simulink library "CassieLibrary"  (R2017b)
settings: Solver=VariableStepAuto  StartTime=0.0  StopTime=10.0  RelTol=1e-3
undefined symbols (not defined in the file): DiagnosticCodes, motorPositions, motorVelocities, X, Y, Z
libraries: sm_lib x50, ComponentLibrary x19, xpcethercatlib x15, CassieLibrary x10, xpcutilitieslib x2, simulink x2, Contact_Forces_Lib x2, nesl_utility x2, slrtlib x1
(part 1 of 3)
settings Model: Creator=Mikhail  LastModifiedBy=jreher

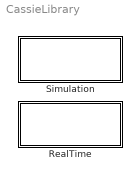
== system CassieLibrary ==
  RealTime : Subsystem
  Simulation : Subsystem

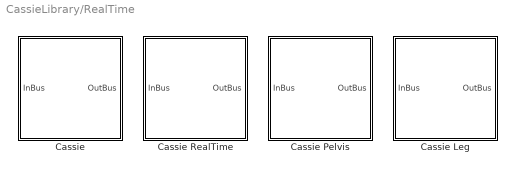
== system CassieLibrary/RealTime ==
  Cassie : Subsystem  InitFcn=|
      | % Import bus definitions
      | CassieModule.importBuses;
      mask Display: image('Cassie.png');
  Cassie Leg : Subsystem  mask{config=Left}
      mask prompts: config "Configuration:"
      mask init:
      | switch config
      |   case 1 % Left
      |     set_param([gcb, '/Hip Roll Drive'], 'ethercatName', 'Left Hip Roll Drive');
      |     set_param([gcb, '/Hip Roll Drive'], 'slaveAddress', '1002');
      |     set_param([gcb, '/Hip Yaw Drive'], 'ethercatName', 'Left Hip Yaw Drive');
      |     set_param([gcb, '/Hip Yaw Drive'], 'slaveAddress', '1003');
      |     set_param([gcb, '/Hip Pitch Drive'], 'ethercatName', 'Left Hip Pitch Drive');
      |     set_param([gcb, '/Hip Pitch Drive'], 'slaveAddress', '1004');
      |     set_param([gcb, '/Knee Drive'], 'ethercatName', 'Left Knee Drive');
      |     set_param([gcb, '/Knee Drive'], 'slaveAddress', '1005');
      |     set_param([gcb, '/Foot Drive'], 'ethercatName', 'Left Foot Drive');
      |     set_param([gcb, '/Foot Drive'], 'slaveAddress', '1006');
      |     set_param([gcb, '/Counter PDO Receive'], 'sig_name', 'Left Leg Medulla.Base Inputs.Counter');
      |     set_param([gcb, '/CPU Load PDO Receive'], 'sig_name', 'Left Leg Medulla.Base Inputs.CPU Load');
      |     set_param([gcb, '/Reed Switch State PDO Receive'], 'sig_name', 'Left Leg Medulla.Misc Inputs.Reed Switch');
      |     set_param([gcb, '/Shin Joint Encoder PDO Receive'], 'sig_name', 'Left Leg Medulla.Misc Inputs.Knee Spring Encoder');
      |     set_param([gcb, '/Tarsus Joint Encoder PDO Receive'], 'sig_name', 'Left Leg Medulla.Misc Inputs.Ankle Joint Encoder');
      |     set_param([gcb, '/Foot Joint Encoder PDO Receive'], 'sig_name', 'Left Leg Medulla.Misc Inputs.Foot Joint Encoder');
      |     set_param([gcb, '/Shin Joint Encoder Gain'], 'Gain', '-1/2^19*2*pi');
      |     set_param([gcb, '/Tarsus Joint Encoder Gain'], 'Gain', '-1/2^19*2*pi');
      |     set_param([gcb, '/Foot Joint Encoder Gain'], 'Gain', '-1/2^13*2*pi');
      |     
      |   case 2 % Right
      |     set_param([gcb, '/Hip Roll Drive'], 'ethercatName', 'Right Hip Roll Drive');
      |     set_param([gcb, '/Hip Roll Drive'], 'slaveAddress', '1008');
      |     set_param([gcb, '/Hip Yaw Drive'], 'ethercatName', 'Right Hip Yaw Drive');
      |     set_param([gcb, '/Hip Yaw Drive'], 'slaveAddress', '1009');
      |     set_param([gcb, '/Hip Pitch Drive'], 'ethercatName', 'Right Hip Pitch Drive');
      |     set_param([gcb, '/Hip Pitch Drive'], 'slaveAddress', '1012');
      |     set_param([gcb, '/Knee Drive'], 'ethercatName', 'Right Knee Drive');
      |     set_param([gcb, '/Knee Drive'], 'slaveAddress', '1011');
      |     set_param([gcb, '/Foot Drive'], 'ethercatName', 'Right Foot Drive');
      |     set_param([gcb, '/Foot Drive'], 'slaveAddress', '1010');
      |     set_param([gcb, '/Counter PDO Receive'], 'sig_name', 'Right Leg Medulla.Base Inputs.Counter');
      |     set_param([gcb, '/CPU Load PDO Receive'], 'sig_name', 'Right Leg Medulla.Base Inputs.CPU Load');
      |     set_param([gcb, '/Reed Switch State PDO Receive'], 'sig_name', 'Right Leg Medulla.Misc Inputs.Reed Switch');
      |     set_param([gcb, '/Shin Joint Encoder PDO Receive'], 'sig_name', 'Right Leg Medulla.Misc Inputs.Knee Spring Encoder');
      |     set_param([gcb, '/Tarsus Joint Encoder PDO Receive'], 'sig_name', 'Right Leg Medulla.Misc Inputs.Ankle Joint Encoder');
      |     set_param([gcb, '/Foot Joint Encoder PDO Receive'], 'sig_name', 'Right Leg Medulla.Misc Inputs.Foot Joint Encoder');
      |     set_param([gcb, '/Shin Joint Encoder Gain'], 'Gain', '1/2^19*2*pi');
      |     set_param([gcb, '/Tarsus Joint Encoder Gain'], 'Gain', '1/2^19*2*pi');
      |     set_param([gcb, '/Foot Joint Encoder Gain'], 'Gain', '1/2^13*2*pi');
      | end % switch
      | 
      | % Check if block is not in library model
      | if ~bdIsLibrary(bdroot)
      |   % Construct discrete filter for velocity estimation
      |   dt = str2num(get_param(bdroot, 'FixedStep'));
      |   filter1 = ButterworthFilter(2);
      |   filter1.setTimeConstant(0.003, dt);
      |   filter2 = BackwardDifferencingFilter(2);
      |   filter2.setSampleTime(dt);
      |   filter3 = Filter(filter1, filter2, 'cascade');
      |   [a, b] = filter3.getCoefficients;
      |   
      |   % Set discrete filter coefficients    
      |   set_param([gcb '/Shin Filter'], 'a', mat2str(a));
      |   set_param([gcb '/Shin Filter'], 'b', mat2str(b));
      |   set_param([gcb '/Tarsus Filter'], 'a', mat2str(a));
      |   set_param([gcb '/Tarsus Filter'], 'b', mat2str(b));
      |   set_param([gcb '/Foot Filter'], 'a', mat2str(a));
      |   set_param([gcb '/Foot Filter'], 'b', mat2str(b));
      | end % if
      settings: PermitHierarchicalResolution=None
      mask TypeOptions config: Left | Right
  Cassie Pelvis : Subsystem
      settings: PermitHierarchicalResolution=None
  Cassie RealTime : Subsystem
      settings: PermitHierarchicalResolution=None
      mask Display: image('Cassie.png');

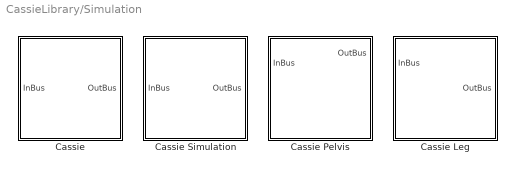
== system CassieLibrary/Simulation ==
  Cassie : Subsystem  InitFcn=|  StartFcn=|  StopFcn=|
      InitFcn=|
      | % Start clock at initialization (used for computing real time performance)
      | initTime = tic;
      | 
      | % Import bus definitions
      | CassieModule.importBuses;
      StartFcn=|
      | % Store build time
      | buildTime = toc(initTime);
      StopFcn=|
      | % Store computation time
      | computationTime = toc(initTime) - buildTime;
      | 
      | % Get simulation time
      | simulationTime = get_param(bdroot, 'SimulationTime');
      | 
      | % Compute real time performance
      | percentRealTime = 100*simulationTime/computationTime;
      | 
      | % Display
      | fprintf('Build time: %0.2f seconds \n', buildTime);
      | fprintf('Simulation time: %0.2f seconds \n', simulationTime);
      | fprintf('Computation time: %0.2f seconds \n', computationTime);
      | fprintf('Performance: %0.2f%% real time \n', percentRealTime);
      mask Display: image('Cassie.png');
  Cassie Leg : Subsystem  mask{config=Right, motorPositions=motorPositions(6:10), motorVelocities=motorVelocities(6:10)}
      mask prompts: config "Configuration:"; motorPositions "Initial Motor Positions (rad):"; motorVelocities "Initial Motor Velocities (rad/s):"
      mask init:
      | d = CassieDescriptor;
      | bodyIndex = @(s, name) find(arrayfun(@(s) isequal(s.name, name), s));
      | 
      | switch config
      |   case 1 % Left
      |     % Hip Roll
      |     b = d(bodyIndex(d, 'left-hip-roll'));
      |     set_param([gcb, '/Hip Roll Solid'], 'ExtGeomFileName', [b.name '.stl']);
      |     set_param([gcb, '/Hip Roll Solid'], 'Mass', mat2str(b.m));
      |     set_param([gcb, '/Hip Roll Solid'], 'CenterOfMass', mat2str(b.c));
      |     set_param([gcb, '/Hip Roll Solid'], 'MomentsOfInertia', mat2str(b.Ic(1:3)));
      |     set_param([gcb, '/Hip Roll Solid'], 'ProductsOfInertia', mat2str(b.Ic(4:6)));
      |     %set_param([gcb, '/Pelvis to Hip Roll'], 'TranslationCartesianOffset', mat2str(b.r));
      |     %set_param([gcb, '/Pelvis to Hip Roll'], 'RotationMatrix', mat2str(b.R));
      |     
      |     % Hip Yaw
      |     b = d(bodyIndex(d, 'left-hip-yaw'));
      |     set_param([gcb, '/Hip Yaw Solid'], 'ExtGeomFileName', [b.name '.stl']);
      |     set_param([gcb, '/Hip Yaw Solid'], 'Mass', mat2str(b.m));
      |     set_param([gcb, '/Hip Yaw Solid'], 'CenterOfMass', mat2str(b.c));
      |     set_param([gcb, '/Hip Yaw Solid'], 'MomentsOfInertia', mat2str(b.Ic(1:3)));
      |     set_param([gcb, '/Hip Yaw Solid'], 'ProductsOfInertia', mat2str(b.Ic(4:6)));
      |     set_param([gcb, '/Hip Roll to Hip Yaw'], 'TranslationCartesianOffset', mat2str(b.r));
      |     set_param([gcb, '/Hip Roll to Hip Yaw'], 'RotationMatrix', mat2str(b.R));
      |     
      |     % Hip Pitch
      |     b = d(bodyIndex(d, 'left-hip-pitch'));
      |     set_param([gcb, '/Hip Pitch Solid'], 'ExtGeomFileName', [b.name '.stl']);
      |     set_param([gcb, '/Hip Pitch Solid'], 'Mass', mat2str(b.m));
      |     set_param([gcb, '/Hip Pitch Solid'], 'CenterOfMass', mat2str(b.c));
      |     set_param([gcb, '/Hip Pitch Solid'], 'MomentsOfInertia', mat2str(b.Ic(1:3)));
      |     set_param([gcb, '/Hip Pitch Solid'], 'ProductsOfInertia', mat2str(b.Ic(4:6)));
      |     set_param([gcb, '/Hip Yaw to Hip Pitch'], 'TranslationCartesianOffset', mat2str(b.r));
      |     set_param([gcb, '/Hip Yaw to Hip Pitch'], 'RotationMatrix', mat2str(b.R));
      |     
      |     % Achilles Rod
      |     b = d(bodyIndex(d, 'left-achilles-rod'));
      |     set_param([gcb, '/Achilles Rod Solid'], 'ExtGeomFileName', [b.name '.stl']);
      |     set_param([gcb, '/Achilles Rod Solid'], 'Mass', mat2str(b.m));
      |     set_param([gcb, '/Achilles Rod Solid'], 'CenterOfMass', mat2str(b.c));
      |     set_param([gcb, '/Achilles Rod Solid'], 'MomentsOfInertia', mat2str(b.Ic(1:3)));
      |     set_param([gcb, '/Achilles Rod Solid'], 'ProductsOfInertia', mat2str(b.Ic(4:6)));
      |     set_param([gcb, '/Hip Pitch to Achilles Rod'], 'TranslationCartesianOffset', mat2str(b.r));
      |     set_param([gcb, '/Hip Pitch to Achilles Rod'], 'RotationMatrix', mat2str(b.R));
      |     
      |     % Knee
      |     b = d(bodyIndex(d, 'left-knee'));
      |     set_param([gcb, '/Knee Solid'], 'ExtGeomFileName', [b.name '.stl']);
      |     set_param([gcb, '/Knee Solid'], 'Mass', mat2str(b.m));
      |     set_param([gcb, '/Knee Solid'], 'CenterOfMass', mat2str(b.c));
      |     set_param([gcb, '/Knee Solid'], 'MomentsOfInertia', mat2str(b.Ic(1:3)));
      |     set_param([gcb, '/Knee Solid'], 'ProductsOfInertia', mat2str(b.Ic(4:6)));
      |     set_param([gcb, '/Hip Pitch to Knee'], 'TranslationCartesianOffset', mat2str(b.r));
      |     set_param([gcb, '/Hip Pitch to Knee'], 'RotationMatrix', mat2str(b.R));
      |     
      |     % Knee Spring
      |     b = d(bodyIndex(d, 'left-knee-spring'));
      |     set_param([gcb, '/Knee Spring Solid'], 'ExtGeomFileName', [b.name '.stl']);
      |     set_param([gcb, '/Knee Spring Solid'], 'Mass', mat2str(b.m));
      |     set_param([gcb, '/Knee Spring Solid'], 'CenterOfMass', mat2str(b.c));
      |     set_param([gcb, '/Knee Spring Solid'], 'MomentsOfInertia', mat2str(b.Ic(1:3)));
      |     set_param([gcb, '/Knee Spring Solid'], 'ProductsOfInertia', mat2str(b.Ic(4:6)));
      |     set_param([gcb, '/Knee to Knee Spring'], 'TranslationCartesianOffset', mat2str(b.r));
      |     set_param([gcb, '/Knee to Knee Spring'], 'RotationMatrix', mat2str(b.R));
      |     
      |     % Shin
      |     b = d(bodyIndex(d, 'left-shin'));
      |     set_param([gcb, '/Shin Solid'], 'ExtGeomFileName', [b.name '.stl']);
      |     set_param([gcb, '/Shin Solid'], 'Mass', mat2str(b.m));
      |     set_param([gcb, '/Shin Solid'], 'CenterOfMass', mat2str(b.c));
      |     set_param([gcb, '/Shin Solid'], 'MomentsOfInertia', mat2str(b.Ic(1:3)));
      |     set_param([gcb, '/Shin Solid'], 'ProductsOfInertia', mat2str(b.Ic(4:6)));
      |     set_param([gcb, '/Knee to Shin'], 'TranslationCartesianOffset', mat2str(b.r));
      |     set_param([gcb, '/Knee to Shin'], 'RotationMatrix', mat2str(b.R));
      |     
      |     % Tarsus
      |     b = d(bodyIndex(d, 'left-tarsus'));
      |     set_param([gcb, '/Tarsus Solid'], 'ExtGeomFileName', [b.name '.stl']);
      |     set_param([gcb, '/Tarsus Solid'], 'Mass', mat2str(b.m));
      |     set_param([gcb, '/Tarsus Solid'], 'CenterOfMass', mat2str(b.c));
      |     set_param([gcb, '/Tarsus Solid'], 'MomentsOfInertia', mat2str(b.Ic(1:3)));
      |     set_param([gcb, '/Tarsus Solid'], 'ProductsOfInertia', mat2str(b.Ic(4:6)));
      |     set_param([gcb, '/Shin to Tarsus'], 'TranslationCartesianOffset', mat2str(b.r));
      |     set_param([gcb, '/Shin to Tarsus'], 'RotationMatrix', mat2str(b.R));
      |     
      |     % Heel Spring
      |     b = d(bodyIndex(d, 'left-heel-spring'));
      |     set_param([gcb, '/Heel Spring Solid'], 'ExtGeomFileName', [b.name '.stl']);
      |     set_param([gcb, '/Heel Spring Solid'], 'Mass', mat2str(b.m));
      |     set_param([gcb, '/Heel Spring Solid'], 'CenterOfMass', mat2str(b.c));
      |     set_param([gcb, '/Heel Spring Solid'], 'MomentsOfInertia', mat2str(b.Ic(1:3)));
      |     set_param([gcb, '/Heel Spring Solid'], 'ProductsOfInertia', mat2str(b.Ic(4:6)));
      |     set_param([gcb, '/Tarsus to Heel Spring'], 'TranslationCartesianOffset', mat2str(b.r));
      |     set_param([gcb, '/Tarsus to Heel Spring'], 'RotationMatrix', mat2str(b.R));
      |     
      |     % Foot Crank
      |     b = d(bodyIndex(d, 'left-foot-crank'));
      |     set_param([gcb, '/Foot Crank Solid'], 'ExtGeomFileName', [b.name '.stl']);
      |     set_param([gcb, '/Foot Crank Solid'], 'Mass', mat2str(b.m));
      |     set_param([gcb, '/Foot Crank Solid'], 'CenterOfMass', mat2str(b.c));
      |     set_param([gcb, '/Foot Crank Solid'], 'MomentsOfInertia', mat2str(b.Ic(1:3)));
      |     set_param([gcb, '/Foot Crank Solid'], 'ProductsOfInertia', mat2str(b.Ic(4:6)));
      |     set_param([gcb, '/Tarsus to Foot Crank'], 'TranslationCartesianOffset', mat2str(b.r));
      |     set_param([gcb, '/Tarsus to Foot Crank'], 'RotationMatrix', mat2str(b.R));
      |     
      |     % Plantar Rod
      |     b = d(bodyIndex(d, 'left-plantar-rod'));
      |     set_param([gcb, '/Plantar Rod Solid'], 'ExtGeomFileName', [b.name '.stl']);
      |     set_param([gcb, '/Plantar Rod Solid'], 'Mass', mat2str(b.m));
      |     set_param([gcb, '/Plantar Rod Solid'], 'CenterOfMass', mat2str(b.c));
      |     set_param([gcb, '/Plantar Rod Solid'], 'MomentsOfInertia', mat2str(b.Ic(1:3)));
      |     set_param([gcb, '/Plantar Rod Solid'], 'ProductsOfInertia', mat2str(b.Ic(4:6)));
      |     set_param([gcb, '/Foot Crank to Plantar Rod'], 'TranslationCartesianOffset', mat2str(b.r));
      |     set_param([gcb, '/Foot Crank to Plantar Rod'], 'RotationMatrix', mat2str(b.R));
      |     
      |     % Foot
      |     b = d(bodyIndex(d, 'left-foot'));
      |     set_param([gcb, '/Foot Solid'], 'ExtGeomFileName', [b.name '.stl']);
      |     set_param([gcb, '/Foot Solid'], 'Mass', mat2str(b.m));
      |     set_param([gcb, '/Foot Solid'], 'CenterOfMass', mat2str(b.c));
      |     set_param([gcb, '/Foot Solid'], 'MomentsOfInertia', mat2str(b.Ic(1:3)));
      |     set_param([gcb, '/Foot Solid'], 'ProductsOfInertia', mat2str(b.Ic(4:6)));
      |     set_param([gcb, '/Tarsus to Foot'], 'TranslationCartesianOffset', mat2str(b.r));
      |     set_param([gcb, '/Tarsus to Foot'], 'RotationMatrix', mat2str(b.R));
      |     
      |     % Foot Pin
      |     %b = d(bodyIndex(d, 'left-foot-pin'));
      |     set_param([gcb, '/Foot to Foot Pin'], 'TranslationCartesianOffset', mat2str([0.055 0 0.00776]));
      |     set_param([gcb, '/Foot to Foot Pin'], 'RotationMatrix', mat2str(eye(3)));
      |     
      |     % Midfoot
      |     %b = d(bodyIndex(d, 'left-mid-foot'));
      |     set_param([gcb, '/Foot to Midfoot'], 'TranslationCartesianOffset', mat2str([0.01762 0.05219 0]));
      |     set_param([gcb, '/Foot to Midfoot'], 'RotationMatrix', mat2str([-0.766044443118978 0 -0.642787609686539;0.642787609686539 0 -0.766044443118978;0 -1 0]));
      |     
      |   case 2 % Right
      |     % Hip Roll
      |     b = d(bodyIndex(d, 'right-hip-roll'));
      |     set_param([gcb, '/Hip Roll Solid'], 'ExtGeomFileName', [b.name '.stl']);
      |     set_param([gcb, '/Hip Roll Solid'], 'Mass', mat2str(b.m));
      |     set_param([gcb, '/Hip Roll Solid'], 'CenterOfMass', mat2str(b.c));
      |     set_param([gcb, '/Hip Roll Solid'], 'MomentsOfInertia', mat2str(b.Ic(1:3)));
      |     set_param([gcb, '/Hip Roll Solid'], 'ProductsOfInertia', mat2str(b.Ic(4:6)));
      |     %set_param([gcb, '/Pelvis to Hip Roll'], 'TranslationCartesianOffset', mat2str(b.r));
      |     %set_param([gcb, '/Pelvis to Hip Roll'], 'RotationMatrix', mat2str(b.R));
      |     
      |     % Hip Yaw
      |     b = d(bodyIndex(d, 'right-hip-yaw'));
      |     set_param([gcb, '/Hip Yaw Solid'], 'ExtGeomFileName', [b.name '.stl']);
      |     set_param([gcb, '/Hip Yaw Solid'], 'Mass', mat2str(b.m));
      |     set_param([gcb, '/Hip Yaw Solid'], 'CenterOfMass', mat2str(b.c));
      |     set_param([gcb, '/Hip Yaw Solid'], 'MomentsOfInertia', mat2str(b.Ic(1:3)));
      |     set_param([gcb, '/Hip Yaw Solid'], 'ProductsOfInertia', mat2str(b.Ic(4:6)));
      |     set_param([gcb, '/Hip Roll to Hip Yaw'], 'TranslationCartesianOffset', mat2str(b.r));
      |     set_param([gcb, '/Hip Roll to Hip Yaw'], 'RotationMatrix', mat2str(b.R));
      |     
      |     % Hip Pitch
      |     b = d(bodyIndex(d, 'right-hip-pitch'));
      |     set_param([gcb, '/Hip Pitch Solid'], 'ExtGeomFileName', [b.name '.stl']);
      |     set_param([gcb, '/Hip Pitch Solid'], 'Mass', mat2str(b.m));
      |     set_param([gcb, '/Hip Pitch Solid'], 'CenterOfMass', mat2str(b.c));
      |     set_param([gcb, '/Hip Pitch Solid'], 'MomentsOfInertia', mat2str(b.Ic(1:3)));
      |     set_param([gcb, '/Hip Pitch Solid'], 'ProductsOfInertia', mat2str(b.Ic(4:6)));
      |     set_param([gcb, '/Hip Yaw to Hip Pitch'], 'TranslationCartesianOffset', mat2str(b.r));
      |     set_param([gcb, '/Hip Yaw to Hip Pitch'], 'RotationMatrix', mat2str(b.R));
      |     
      |     % Achilles Rod
      |     b = d(bodyIndex(d, 'right-achilles-rod'));
      |     set_param([gcb, '/Achilles Rod Solid'], 'ExtGeomFileName', [b.name '.stl']);
      |     set_param([gcb, '/Achilles Rod Solid'], 'Mass', mat2str(b.m));
      |     set_param([gcb, '/Achilles Rod Solid'], 'CenterOfMass', mat2str(b.c));
      |     set_param([gcb, '/Achilles Rod Solid'], 'MomentsOfInertia', mat2str(b.Ic(1:3)));
      |     set_param([gcb, '/Achilles Rod Solid'], 'ProductsOfInertia', mat2str(b.Ic(4:6)));
      |     set_param([gcb, '/Hip Pitch to Achilles Rod'], 'TranslationCartesianOffset', mat2str(b.r));
      |     set_param([gcb, '/Hip Pitch to Achilles Rod'], 'RotationMatrix', mat2str(b.R));
      |     
      |     % Knee
      |     b = d(bodyIndex(d, 'right-knee'));
      |     set_param([gcb, '/Knee Solid'], 'ExtGeomFileName', [b.name '.stl']);
      |     set_param([gcb, '/Knee Solid'], 'Mass', mat2str(b.m));
      |     set_param([gcb, '/Knee Solid'], 'CenterOfMass', mat2str(b.c));
      |     set_param([gcb, '/Knee Solid'], 'MomentsOfInertia', mat2str(b.Ic(1:3)));
      |     set_param([gcb, '/Knee Solid'], 'ProductsOfInertia', mat2str(b.Ic(4:6)));
      |     set_param([gcb, '/Hip Pitch to Knee'], 'TranslationCartesianOffset', mat2str(b.r));
      |     set_param([gcb, '/Hip Pitch to Knee'], 'RotationMatrix', mat2str(b.R));
      |     
      |     % Knee Spring
      |     b = d(bodyIndex(d, 'right-knee-spring'));
      |     set_param([gcb, '/Knee Spring Solid'], 'ExtGeomFileName', [b.name '.stl']);
      |     set_param([gcb, '/Knee Spring Solid'], 'Mass', mat2str(b.m));
      |     set_param([gcb, '/Knee Spring Solid'], 'CenterOfMass', mat2str(b.c));
      |     set_param([gcb, '/Knee Spring Solid'], 'MomentsOfInertia', mat2str(b.Ic(1:3)));
      |     set_param([gcb, '/Knee Spring Solid'], 'ProductsOfInertia', mat2str(b.Ic(4:6)));
      |     set_param([gcb, '/Knee to Knee Spring'], 'TranslationCartesianOffset', mat2str(b.r));
      |     set_param([gcb, '/Knee to Knee Spring'], 'RotationMatrix', mat2str(b.R));
      |     
      |     % Shin
      |     b = d(bodyIndex(d, 'right-shin'));
      |     set_param([gcb, '/Shin Solid'], 'ExtGeomFileName', [b.name '.stl']);
      |     set_param([gcb, '/Shin Solid'], 'Mass', mat2str(b.m));
      |     set_param([gcb, '/Shin Solid'], 'CenterOfMass', mat2str(b.c));
      |     set_param([gcb, '/Shin Solid'], 'MomentsOfInertia', mat2str(b.Ic(1:3)));
      |     set_param([gcb, '/Shin Solid'], 'ProductsOfInertia', mat2str(b.Ic(4:6)));
      |     set_param([gcb, '/Knee to Shin'], 'TranslationCartesianOffset', mat2str(b.r));
      |     set_param([gcb, '/Knee to Shin'], 'RotationMatrix', mat2str(b.R));
      |     
      |     % Tarsus
      |     b = d(bodyIndex(d, 'right-tarsus'));
      |     set_param([gcb, '/Tarsus Solid'], 'ExtGeomFileName', [b.name '.stl']);
      |     set_param([gcb, '/Tarsus Solid'], 'Mass', mat2str(b.m));
      |     set_param([gcb, '/Tarsus Solid'], 'CenterOfMass', mat2str(b.c));
      |     set_param([gcb, '/Tarsus Solid'], 'MomentsOfInertia', mat2str(b.Ic(1:3)));
      |     set_param([gcb, '/Tarsus Solid'], 'ProductsOfInertia', mat2str(b.Ic(4:6)));
      |     set_param([gcb, '/Shin to Tarsus'], 'TranslationCartesianOffset', mat2str(b.r));
      |     set_param([gcb, '/Shin to Tarsus'], 'RotationMatrix', mat2str(b.R));
      |     
      |     % Heel Spring
      |     b = d(bodyIndex(d, 'right-heel-spring'));
      |     set_param([gcb, '/Heel Spring Solid'], 'ExtGeomFileName', [b.name '.stl']);
      |     set_param([gcb, '/Heel Spring Solid'], 'Mass', mat2str(b.m));
      |     set_param([gcb, '/Heel Spring Solid'], 'CenterOfMass', mat2str(b.c));
      |     set_param([gcb, '/Heel Spring Solid'], 'MomentsOfInertia', mat2str(b.Ic(1:3)));
      |     set_param([gcb, '/Heel Spring Solid'], 'ProductsOfInertia', mat2str(b.Ic(4:6)));
      |     set_param([gcb, '/Tarsus to Heel Spring'], 'TranslationCartesianOffset', mat2str(b.r));
      |     set_param([gcb, '/Tarsus to Heel Spring'], 'RotationMatrix', mat2str(b.R));
      |     
      |     % Foot Crank
      |     b = d(bodyIndex(d, 'right-foot-crank'));
      |     set_param([gcb, '/Foot Crank Solid'], 'ExtGeomFileName', [b.name '.stl']);
      |     set_param([gcb, '/Foot Crank Solid'], 'Mass', mat2str(b.m));
      |     set_param([gcb, '/Foot Crank Solid'], 'CenterOfMass', mat2str(b.c));
      |     set_param([gcb, '/Foot Crank Solid'], 'MomentsOfInertia', mat2str(b.Ic(1:3)));
      |     set_param([gcb, '/Foot Crank Solid'], 'ProductsOfInertia', mat2str(b.Ic(4:6)));
      |     set_param([gcb, '/Tarsus to Foot Crank'], 'TranslationCartesianOffset', mat2str(b.r));
      |     set_param([gcb, '/Tarsus to Foot Crank'], 'RotationMatrix', mat2str(b.R));
      |     
      |     % Plantar Rod
      |     b = d(bodyIndex(d, 'right-plantar-rod'));
      |     set_param([gcb, '/Plantar Rod Solid'], 'ExtGeomFileName', [b.name '.stl']);
      |     set_param([gcb, '/Plantar Rod Solid'], 'Mass', mat2str(b.m));
      |     set_param([gcb, '/Plantar Rod Solid'], 'CenterOfMass', mat2str(b.c));
      |     set_param([gcb, '/Plantar Rod Solid'], 'MomentsOfInertia', mat2str(b.Ic(1:3)));
      |     set_param([gcb, '/Plantar Rod Solid'], 'ProductsOfInertia', mat2str(b.Ic(4:6)));
      |     set_param([gcb, '/Foot Crank to Plantar Rod'], 'TranslationCartesianOffset', mat2str(b.r));
      |     set_param([gcb, '/Foot Crank to Plantar Rod'], 'RotationMatrix', mat2str(b.R));
      |     
      |     % Foot
      |     b = d(bodyIndex(d, 'right-foot'));
      |     set_param([gcb, '/Foot Solid'], 'ExtGeomFileName', [b.name '.stl']);
      |     set_param([gcb, '/Foot Solid'], 'Mass', mat2str(b.m));
      |     set_param([gcb, '/Foot Solid'], 'CenterOfMass', mat2str(b.c));
      |     set_param([gcb, '/Foot Solid'], 'MomentsOfInertia', mat2str(b.Ic(1:3)));
      |     set_param([gcb, '/Foot Solid'], 'ProductsOfInertia', mat2str(b.Ic(4:6)));
      |     set_param([gcb, '/Tarsus to Foot'], 'TranslationCartesianOffset', mat2str(b.r));
      |     set_param([gcb, '/Tarsus to Foot'], 'RotationMatrix', mat2str(b.R));
      |     
      |     % Foot Pin
      |     %b = d(bodyIndex(d, 'right-foot-pin'));
      |     set_param([gcb, '/Foot to Foot Pin'], 'TranslationCartesianOffset', mat2str([0.055 0 -0.00776]));
      |     set_param([gcb, '/Foot to Foot Pin'], 'RotationMatrix', mat2str(eye(3)));
      |     
      |     % Midfoot
      |     %b = d(bodyIndex(d, 'right-mid-foot'));
      |     set_param([gcb, '/Foot to Midfoot'], 'TranslationCartesianOffset', mat2str([0.01762 0.05219 0]));
      |     set_param([gcb, '/Foot to Midfoot'], 'RotationMatrix', mat2str([-0.766044443118978 0 -0.642787609686539;0.642787609686539 0 -0.766044443118978;0 -1 0]));
      | end % switch
      | 
      | % Check if block is not in library model
      | if ~bdIsLibrary(bdroot)
      |   % Construct discrete filter for velocity estimation
      |   dt = str2num(get_param(bdroot, 'FixedStep'));
      |   filter1 = ButterworthFilter(2);
      |   filter1.setTimeConstant(0.003, dt);
      |   filter2 = BackwardDifferencingFilter(2);
      |   filter2.setSampleTime(dt);
      |   filter3 = Filter(filter1, filter2, 'cascade');
      |   [a, b] = filter3.getCoefficients;
      |   
      |   % Set discrete filter coefficients    
      |   set_param([gcb '/Shin Filter'], 'a', mat2str(a));
      |   set_param([gcb '/Shin Filter'], 'b', mat2str(b));
      |   set_param([gcb '/Tarsus Filter'], 'a', mat2str(a));
      |   set_param([gcb '/Tarsus Filter'], 'b', mat2str(b));
      |   set_param([gcb '/Foot Filter'], 'a', mat2str(a));
      |   set_param([gcb '/Foot Filter'], 'b', mat2str(b));
      | end % if
      mask TypeOptions config: Left | Right
  Cassie Pelvis : Subsystem
  Cassie Simulation : Subsystem
      mask Display: image('Cassie.png');

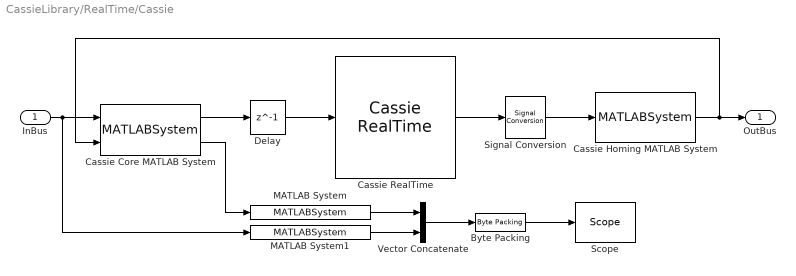
== system CassieLibrary/RealTime/Cassie ==
  InBus : Inport  OutDataTypeStr=Bus: CassieUserInBus
  "Byte Packing " : xpcutilitieslib/Byte Packing   MaskPackedDataType=double  MaskUnpackedDataTypes={'uint8'}  MaskAlignment=1
  Cassie Core MATLAB System : MATLABSystem  System=CassieCore  SimulateUsing=Code generation
      mask Type: CassieCore
      mask Display: disp('CassieCore');
  Cassie Homing MATLAB System : MATLABSystem  System=CassieHoming  SimulateUsing=Code generation
      mask Type: CassieHoming
      mask Display: disp('CassieHoming');
  Cassie RealTime : CassieLibrary/RealTime/Cassie RealTime  SystemSampleTime=-1
  Delay : Delay  DelayLength=1
  MATLAB System : MATLABSystem  System=CassieOutBusToBytes  SimulateUsing=Code generation
      mask Type: CassieOutBusToBytes
      mask Display: disp('CassieOutBusToBytes');
  MATLAB System1 : MATLABSystem  System=CassieUserInBusToBytes  SimulateUsing=Code generation
      mask Type: CassieUserInBusToBytes
      mask Display: disp('CassieUserInBusToBytes');
  "Scope " : slrtlib/Displays and Logging/Scope   scopeno=1  scopetype=File  autostart=on  viewmode=Graphical redraw  formatstr='%15.6f'  grid=on  ylimits=[0,0]  nosamples=250  noprepostsamples=0  interleave=1  triggermode=FreeRun  triggersignal=1  trigsignalfromport=off  triggerlevel=0.0  triggerslope=Either  triggerscope=1  triggersample=0  filename=cassie<%>.dat  mode=Commit  writesize=4096  autorestart=on  dynamicfilemode=on  maxwritefilesize=1024^3
  Signal Conversion : SignalConversion  ConversionOutput=Nonvirtual bus  OutDataTypeStr=Bus: CassieOutBus  OverrideOpt=off
  Vector Concatenate : Concatenate
  OutBus : Outport  OutDataTypeStr=Bus: CassieOutBus
  wires:
  Cassie RealTime/1 -> Signal Conversion/1
  InBus/1 -> MATLAB System1/1, Cassie Core MATLAB System/1
  Signal Conversion/1 -> Cassie Homing MATLAB System/1
  Cassie Homing MATLAB System/1 -> Cassie Core MATLAB System/2, OutBus/1
  MATLAB System/1 -> Vector Concatenate/1
  Vector Concatenate/1 -> "Byte Packing "/1
  MATLAB System1/1 -> Vector Concatenate/2
  "Byte Packing "/1 -> "Scope "/1
  Cassie Core MATLAB System/2 -> MATLAB System/1
  Cassie Core MATLAB System/1 -> Delay/1
  Delay/1 -> Cassie RealTime/1

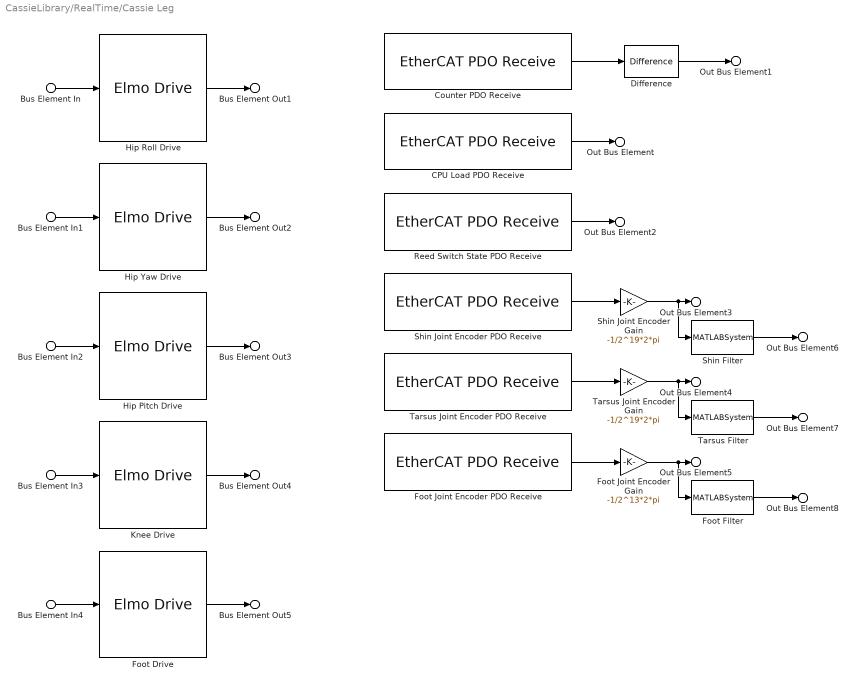
== system CassieLibrary/RealTime/Cassie Leg ==
  Bus Element In : Inport  PortName=InBus  Element=hipRollDrive
  Bus Element In1 : Inport  PortName=InBus  Element=hipYawDrive
  Bus Element In2 : Inport  PortName=InBus  Element=hipPitchDrive
  Bus Element In3 : Inport  PortName=InBus  Element=kneeDrive
  Bus Element In4 : Inport  PortName=InBus  Element=footDrive
  CPU Load PDO Receive : xpcethercatlib/EtherCAT PDO Receive  Priority=2  sig_name=Left Leg Medulla.Base Inputs.CPU Load  sig_offset=600  sig_type=uint16  type_size=16  sig_dim=1  device_id=0  sample_time=0.000500
      settings: SourceProductName=Simulink Real-Time  SourceProductBaseCode=XP
  Counter PDO Receive : xpcethercatlib/EtherCAT PDO Receive  Priority=2  sig_name=Left Leg Medulla.Base Inputs.Counter  sig_offset=592  sig_type=uint8  type_size=8  sig_dim=1  device_id=0  sample_time=0.000500
      settings: SourceProductName=Simulink Real-Time  SourceProductBaseCode=XP
  Difference : simulink/Discrete/Difference  ICPrevInput=0.0  OutMin=[]  OutMax=[]  OutDataType=fixdt(1, 16)  OutScaling=2^-10  DoSatur=off
  Foot Drive : ComponentLibrary/RealTime/Elmo Drive  ethercatName=Left Foot Drive  slaveAddress=1006  gearRatio=50  torqueConstant=0.057  encoderCounts=2^19  peakCurrentLimit=19.74
  Foot Filter : MATLABSystem  System=FilterSystem  a=[]  b=[]  SimulateUsing=Code generation
      mask Type: FilterSystem
      mask Display: disp('Filter');
  Foot Joint Encoder Gain : Gain  Gain=-1/2^13*2*pi  ParamDataTypeStr=double  OutDataTypeStr=double
  Foot Joint Encoder PDO Receive : xpcethercatlib/EtherCAT PDO Receive  Priority=2  sig_name=Left Leg Medulla.Misc Inputs.Foot Joint Encoder  sig_offset=1936  sig_type=int32  type_size=32  sig_dim=1  device_id=0  sample_time=0.000500
      settings: SourceProductName=Simulink Real-Time  SourceProductBaseCode=XP
  Hip Pitch Drive : ComponentLibrary/RealTime/Elmo Drive  ethercatName=Left Hip Pitch Drive  slaveAddress=1004  gearRatio=16  torqueConstant=0.27  encoderCounts=2^13  peakCurrentLimit=50
  Hip Roll Drive : ComponentLibrary/RealTime/Elmo Drive  ethercatName=Left Hip Roll Drive  slaveAddress=1002  gearRatio=25  torqueConstant=0.13  encoderCounts=2^13  peakCurrentLimit=43.27
  Hip Yaw Drive : ComponentLibrary/RealTime/Elmo Drive  ethercatName=Left Hip Yaw Drive  slaveAddress=1003  gearRatio=25  torqueConstant=0.13  encoderCounts=2^13  peakCurrentLimit=43.27
  Knee Drive : ComponentLibrary/RealTime/Elmo Drive  ethercatName=Left Knee Drive  slaveAddress=1005  gearRatio=16  torqueConstant=0.27  encoderCounts=2^13  peakCurrentLimit=50
  Reed Switch State PDO Receive : xpcethercatlib/EtherCAT PDO Receive  Priority=2  sig_name=Left Leg Medulla.Misc Inputs.Reed Switch  sig_offset=1968  sig_type=boolean  type_size=1  sig_dim=1  device_id=0  sample_time=0.000500
      settings: SourceProductName=Simulink Real-Time  SourceProductBaseCode=XP
  Shin Filter : MATLABSystem  System=FilterSystem  a=[]  b=[]  SimulateUsing=Code generation
      mask Type: FilterSystem
      mask Display: disp('Filter');
  Shin Joint Encoder Gain : Gain  Gain=-1/2^19*2*pi  ParamDataTypeStr=double  OutDataTypeStr=double
  Shin Joint Encoder PDO Receive : xpcethercatlib/EtherCAT PDO Receive  Priority=2  sig_name=Left Leg Medulla.Misc Inputs.Knee Spring Encoder  sig_offset=1872  sig_type=int32  type_size=32  sig_dim=1  device_id=0  sample_time=0.000500
      settings: SourceProductName=Simulink Real-Time  SourceProductBaseCode=XP
  Tarsus Filter : MATLABSystem  System=FilterSystem  a=[]  b=[]  SimulateUsing=Code generation
      mask Type: FilterSystem
      mask Display: disp('Filter');
  Tarsus Joint Encoder Gain : Gain  Gain=-1/2^19*2*pi  ParamDataTypeStr=double  OutDataTypeStr=double
  Tarsus Joint Encoder PDO Receive : xpcethercatlib/EtherCAT PDO Receive  Priority=2  sig_name=Left Leg Medulla.Misc Inputs.Ankle Joint Encoder  sig_offset=1904  sig_type=int32  type_size=32  sig_dim=1  device_id=0  sample_time=0.000500
      settings: SourceProductName=Simulink Real-Time  SourceProductBaseCode=XP
  Bus Element Out1 : Outport  PortName=OutBus  Element=hipRollDrive
  Bus Element Out2 : Outport  PortName=OutBus  Element=hipYawDrive
  Bus Element Out3 : Outport  PortName=OutBus  Element=hipPitchDrive
  Bus Element Out4 : Outport  PortName=OutBus  Element=kneeDrive
  Bus Element Out5 : Outport  PortName=OutBus  Element=footDrive
  Out Bus Element3 : Outport  PortName=OutBus  Element=shinJoint.position
  Out Bus Element6 : Outport  PortName=OutBus  Element=shinJoint.velocity
  Out Bus Element4 : Outport  PortName=OutBus  Element=tarsusJoint.position
  Out Bus Element7 : Outport  PortName=OutBus  Element=tarsusJoint.velocity
  Out Bus Element5 : Outport  PortName=OutBus  Element=footJoint.position
  Out Bus Element8 : Outport  PortName=OutBus  Element=footJoint.velocity
  Out Bus Element1 : Outport  PortName=OutBus  Element=medullaCounter
  Out Bus Element : Outport  PortName=OutBus  Element=medullaCpuLoad
  Out Bus Element2 : Outport  PortName=OutBus  Element=reedSwitchState
  wires:
  Hip Roll Drive/1 -> Bus Element Out1/1
  Hip Yaw Drive/1 -> Bus Element Out2/1
  Hip Pitch Drive/1 -> Bus Element Out3/1
  Knee Drive/1 -> Bus Element Out4/1
  Foot Drive/1 -> Bus Element Out5/1
  Bus Element In/1 -> Hip Roll Drive/1
  Bus Element In1/1 -> Hip Yaw Drive/1
  Bus Element In2/1 -> Hip Pitch Drive/1
  Bus Element In3/1 -> Knee Drive/1
  Bus Element In4/1 -> Foot Drive/1
  CPU Load PDO Receive/1 -> Out Bus Element/1
  Reed Switch State PDO Receive/1 -> Out Bus Element2/1
  Counter PDO Receive/1 -> Difference/1
  Tarsus Joint Encoder PDO Receive/1 -> Tarsus Joint Encoder Gain/1
  Difference/1 -> Out Bus Element1/1
  Foot Joint Encoder Gain/1 -> Foot Filter/1, Out Bus Element5/1
  Shin Joint Encoder PDO Receive/1 -> Shin Joint Encoder Gain/1
  Shin Joint Encoder Gain/1 -> Shin Filter/1, Out Bus Element3/1
  Foot Joint Encoder PDO Receive/1 -> Foot Joint Encoder Gain/1
  Tarsus Joint Encoder Gain/1 -> Tarsus Filter/1, Out Bus Element4/1
  Shin Filter/1 -> Out Bus Element6/1
  Tarsus Filter/1 -> Out Bus Element7/1
  Foot Filter/1 -> Out Bus Element8/1

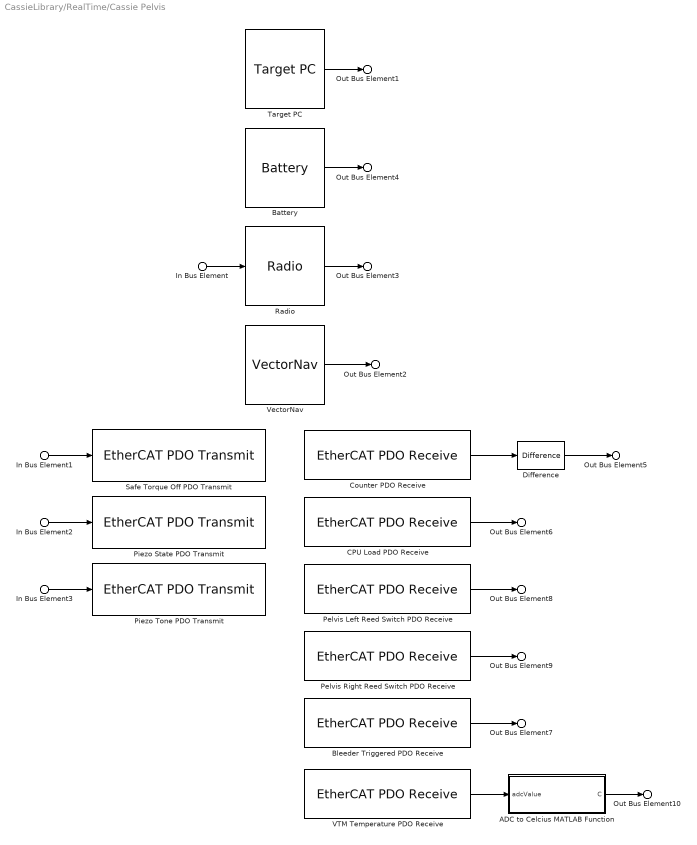
== system CassieLibrary/RealTime/Cassie Pelvis ==
  In Bus Element : Inport  PortName=InBus  Element=radio
  In Bus Element1 : Inport  PortName=InBus  Element=sto
  In Bus Element2 : Inport  PortName=InBus  Element=piezoState
  In Bus Element3 : Inport  PortName=InBus  Element=piezoTone
  ADC to Celcius MATLAB Function : MATLAB Function  TreatAsAtomicUnit=on
  Battery : ComponentLibrary/RealTime/Battery  SystemSampleTime=-1
  Bleeder Triggered PDO Receive : xpcethercatlib/EtherCAT PDO Receive  Priority=2  sig_name=Pelvis Medulla.Misc Inputs.Bleeder State  sig_offset=1888  sig_type=boolean  type_size=1  sig_dim=1  device_id=0  sample_time=0.000500
      settings: SourceProductName=Simulink Real-Time  SourceProductBaseCode=XP
  CPU Load PDO Receive : xpcethercatlib/EtherCAT PDO Receive  Priority=2  sig_name=Pelvis Medulla.Base Inputs.CPU Load  sig_offset=664  sig_type=uint16  type_size=16  sig_dim=1  device_id=0  sample_time=0.000500
      settings: SourceProductName=Simulink Real-Time  SourceProductBaseCode=XP
  Counter PDO Receive : xpcethercatlib/EtherCAT PDO Receive  Priority=2  sig_name=Pelvis Medulla.Base Inputs.Counter  sig_offset=656  sig_type=uint8  type_size=8  sig_dim=1  device_id=0  sample_time=0.000500
      settings: SourceProductName=Simulink Real-Time  SourceProductBaseCode=XP
  Difference : simulink/Discrete/Difference  ICPrevInput=0.0  OutMin=[]  OutMax=[]  OutDataType=fixdt(1, 16)  OutScaling=2^-10  DoSatur=off
  Pelvis Left Reed Switch PDO Receive : xpcethercatlib/EtherCAT PDO Receive  Priority=2  sig_name=Pelvis Medulla.Misc Inputs.Left Reed Switch State  sig_offset=1890  sig_type=boolean  type_size=1  sig_dim=1  device_id=0  sample_time=0.000500
      settings: SourceProductName=Simulink Real-Time  SourceProductBaseCode=XP
  Pelvis Right Reed Switch PDO Receive : xpcethercatlib/EtherCAT PDO Receive  Priority=2  sig_name=Pelvis Medulla.Misc Inputs.Right Reed Switch State  sig_offset=1889  sig_type=boolean  type_size=1  sig_dim=1  device_id=0  sample_time=0.000500
      settings: SourceProductName=Simulink Real-Time  SourceProductBaseCode=XP
  Piezo State PDO Transmit : xpcethercatlib/EtherCAT PDO Transmit   Priority=3  sig_name=Pelvis Medulla.Misc Outputs.Piezo State  sig_offset=881  sig_type=boolean  type_size=1  sig_dim=1  device_id=0  sample_time=0.000500
      settings: SourceProductName=Simulink Real-Time  SourceProductBaseCode=XP
  Piezo Tone PDO Transmit : xpcethercatlib/EtherCAT PDO Transmit   Priority=3  sig_name=Pelvis Medulla.Misc Outputs.Piezo Tone  sig_offset=888  sig_type=uint8  type_size=8  sig_dim=1  device_id=0  sample_time=0.000500
      settings: SourceProductName=Simulink Real-Time  SourceProductBaseCode=XP
  Radio : ComponentLibrary/RealTime/Radio  SystemSampleTime=-1
  Safe Torque Off PDO Transmit : xpcethercatlib/EtherCAT PDO Transmit   Priority=3  sig_name=Pelvis Medulla.Misc Outputs.Medulla STO  sig_offset=880  sig_type=boolean  type_size=1  sig_dim=1  device_id=0  sample_time=0.000500
      settings: SourceProductName=Simulink Real-Time  SourceProductBaseCode=XP
  Target PC : ComponentLibrary/RealTime/Target PC  config_file=cassie-v3-eni.xml  pci_bus=4  pci_slot=0  pci_function=0
  VTM Temperature PDO Receive : xpcethercatlib/EtherCAT PDO Receive  Priority=2  sig_name=Pelvis Medulla.Misc Inputs.VTM Temperature  sig_offset=1896  sig_type=int16  type_size=16  sig_dim=1  device_id=0  sample_time=0.000500
      settings: SourceProductName=Simulink Real-Time  SourceProductBaseCode=XP
  VectorNav : ComponentLibrary/RealTime/VectorNav  preRotationMatrix=[1, 0, 0; 0, -1, 0; 0, 0, -1]  postRotationMatrix=[1, 0, 0; 0, -1, 0; 0, 0, -1]
  Out Bus Element1 : Outport  PortName=OutBus  Element=targetPc
  Out Bus Element4 : Outport  PortName=OutBus  Element=battery
  Out Bus Element3 : Outport  PortName=OutBus  Element=radio
  Out Bus Element2 : Outport  PortName=OutBus  Element=vectorNav
  Out Bus Element5 : Outport  PortName=OutBus  Element=medullaCounter
  Out Bus Element6 : Outport  PortName=OutBus  Element=medullaCpuLoad
  Out Bus Element7 : Outport  PortName=OutBus  Element=bleederState
  Out Bus Element8 : Outport  PortName=OutBus  Element=leftReedSwitchState
  Out Bus Element9 : Outport  PortName=OutBus  Element=rightReedSwitchState
  Out Bus Element10 : Outport  PortName=OutBus  Element=vtmTemperature
  wires:
  Target PC/1 -> Out Bus Element1/1
  In Bus Element1/1 -> Safe Torque Off PDO Transmit/1
  VTM Temperature PDO Receive/1 -> ADC to Celcius MATLAB Function/1(adcValue)
  Difference/1 -> Out Bus Element5/1
  ADC to Celcius MATLAB Function/1(C) -> Out Bus Element10/1
  Battery/1 -> Out Bus Element4/1
  In Bus Element2/1 -> Piezo State PDO Transmit/1
  Pelvis Right Reed Switch PDO Receive/1 -> Out Bus Element9/1
  In Bus Element/1 -> Radio/1
  Bleeder Triggered PDO Receive/1 -> Out Bus Element7/1
  Radio/1 -> Out Bus Element3/1
  Counter PDO Receive/1 -> Difference/1
  VectorNav/1 -> Out Bus Element2/1
  Pelvis Left Reed Switch PDO Receive/1 -> Out Bus Element8/1
  In Bus Element3/1 -> Piezo Tone PDO Transmit/1
  CPU Load PDO Receive/1 -> Out Bus Element6/1

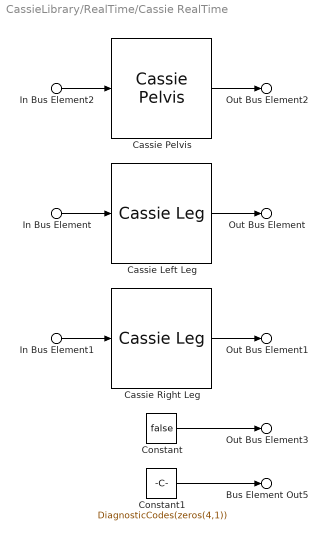
== system CassieLibrary/RealTime/Cassie RealTime ==
  In Bus Element : Inport  PortName=InBus  Element=leftLeg
  In Bus Element1 : Inport  PortName=InBus  Element=rightLeg
  In Bus Element2 : Inport  PortName=InBus  Element=pelvis
  Cassie Left Leg : CassieLibrary/RealTime/Cassie Leg  config=Left
  Cassie Pelvis : CassieLibrary/RealTime/Cassie Pelvis
  Cassie Right Leg : CassieLibrary/RealTime/Cassie Leg  config=Right
  Constant : Constant  Value=false
  Constant1 : Constant  Value=DiagnosticCodes(zeros(4,1))
  Out Bus Element2 : Outport  PortName=OutBus  Element=pelvis
  Out Bus Element : Outport  PortName=OutBus  Element=leftLeg
  Out Bus Element1 : Outport  PortName=OutBus  Element=rightLeg
  Out Bus Element3 : Outport  PortName=OutBus  Element=isCalibrated
  Bus Element Out5 : Outport  PortName=OutBus  Element=messages
  wires:
  Cassie Left Leg/1 -> Out Bus Element/1
  Cassie Right Leg/1 -> Out Bus Element1/1
  In Bus Element/1 -> Cassie Left Leg/1
  In Bus Element1/1 -> Cassie Right Leg/1
  In Bus Element2/1 -> Cassie Pelvis/1
  Cassie Pelvis/1 -> Out Bus Element2/1
  Constant/1 -> Out Bus Element3/1
  Constant1/1 -> Bus Element Out5/1

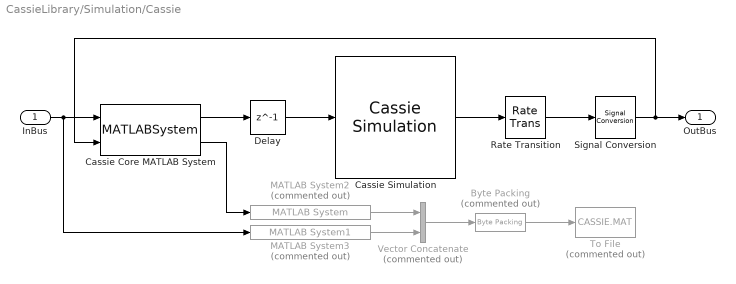
== system CassieLibrary/Simulation/Cassie ==
  InBus : Inport  OutDataTypeStr=Bus: CassieUserInBus
  "Byte Packing " : xpcutilitieslib/Byte Packing   Commented=on  MaskPackedDataType=double  MaskUnpackedDataTypes={'uint8'}  MaskAlignment=1
  Cassie Core MATLAB System : MATLABSystem  System=CassieCoreSim  SimulateUsing=Code generation
      mask Type: CassieCoreSim
      mask Display: disp('CassieCoreSim');
  Cassie Simulation : CassieLibrary/Simulation/Cassie Simulation  SystemSampleTime=-1
  Delay : Delay  DelayLength=1
  MATLAB System2 : CassieLibrary/RealTime/Cassie/MATLAB System  Commented=on  SimulateUsing=Code generation
  MATLAB System3 : CassieLibrary/RealTime/Cassie/MATLAB System1  Commented=on  SimulateUsing=Code generation
  Rate Transition : RateTransition  OutPortSampleTime=0.0005
  Signal Conversion : SignalConversion  ConversionOutput=Nonvirtual bus  OutDataTypeStr=Bus: CassieOutBus  OverrideOpt=off
  To File : ToFile  Commented=on  Filename=CASSIE.MAT  MatrixName=data
  Vector Concatenate : Concatenate  Commented=on
  OutBus : Outport  OutDataTypeStr=Bus: CassieOutBus
  wires:
  Cassie Core MATLAB System/1 -> Delay/1
  Delay/1 -> Cassie Simulation/1
  Rate Transition/1 -> Signal Conversion/1
  Cassie Simulation/1 -> Rate Transition/1
  Vector Concatenate/1 -> "Byte Packing "/1
  InBus/1 -> MATLAB System3/1, Cassie Core MATLAB System/1
  "Byte Packing "/1 -> To File/1
  Signal Conversion/1 -> OutBus/1, Cassie Core MATLAB System/2
  MATLAB System3/1 -> Vector Concatenate/2
  MATLAB System2/1 -> Vector Concatenate/1
  Cassie Core MATLAB System/2 -> MATLAB System2/1
